simulink model "open_loop_model_compare"  (R2022b)
settings: Solver=ode45  StartTime=0.0  StopTime=5  FixedStep=0.01  RelTol=1e-3  EnableMultiTasking=on
settings Model: Creator=cpmcclel  LastModifiedBy=kaiwe
settings SolverCC: AlgebraicLoopSolver=TrustRegion
settings DataIOCC: LimitDataPoints=on  SaveFormat=Array  ReturnWorkspaceOutputs=off
settings OptimizationCC: LifeSpan=inf
settings DebuggingCC: SolverPrmCheckMsg=warning  UnconnectedInputMsg=warning  UnconnectedOutputMsg=warning  UnconnectedLineMsg=warning  SFUnexpectedBacktrackingDiag=warning  SFNoUnconditionalDefaultTransitionDiag=warning  SFExecutionAtInitializationDiag=none  SFMachineParentedDataDiag=warning  ArithmeticOperatorsInVariantConditions=warning
settings HardwareCC: ProdBitPerPointer=32  ProdBitPerSizeT=32  ProdBitPerPtrDiffT=32  ProdLargestAtomicFloat=None  ProdIntDivRoundTo=Undefined  ProdEndianess=Unspecified  ProdWordSize=32  ProdHWDeviceType=32-bit Generic
settings ModelReferenceCC: EnableRefExpFcnMdlSchedulingChecks=on  PropagateSignalLabelsOutOfModel=off
settings SFSimCC: SimUseLocalCustomCode=off  CustomCodeUndefinedFunction=UseInterfaceOnly
settings RTWCC: RTWUseLocalCustomCode=off
settings CodeAppCC: StateflowObjectComments=on
settings GRTTargetCC: TargetLangStandard=C89/C90 (ANSI)
settings ConfigComp: CovMetricSettings=dw  CovSaveCumulativeToWorkspaceVar=on  CovSaveSingleToWorkspaceVar=on  CovExternalEMLEnable=off  CovSFcnEnable=off

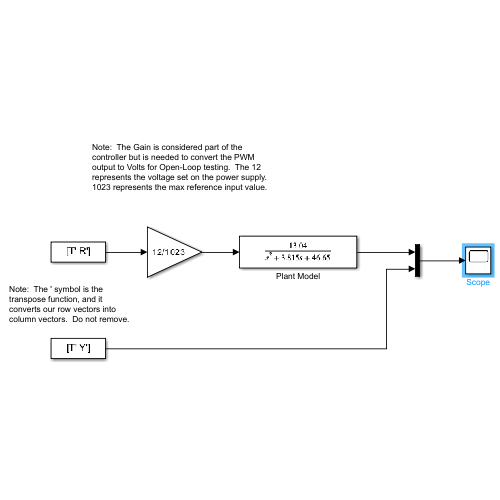
[thumbnail: Simulink's stored preview of the top-level diagram]
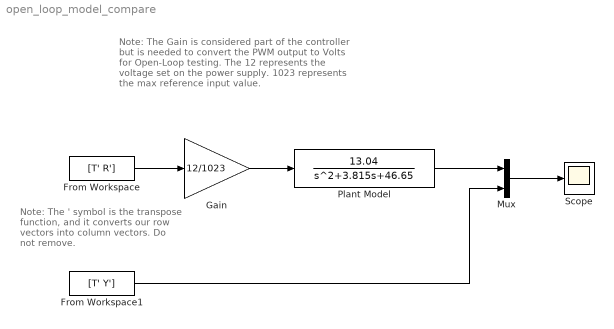
== system open_loop_model_compare ==
  note: Note: The Gain is considered part of the controller but is needed to convert the PWM output to Volts for Open-Loop testing. The 12 represents the voltage set on the power supply. 1023 represents the max reference input value.
  note: Note: The ' symbol is the transpose function, and it converts our row vectors into column vectors. Do not remove.
  From Workspace : FromWorkspace  VariableName=[T' R']  SampleTime=.01
  From Workspace1 : FromWorkspace  VariableName=[T' Y']  SampleTime=-1
  Gain : Gain  Gain=12/1023
  Mux : Mux  Inputs=2
  Plant Model : TransferFcn  Numerator=[13.04]  Denominator=[1 3.815 46.65]
  Scope : Scope
  wires:
  From Workspace/1 -> Gain/1
  Mux/1 -> Scope/1
  From Workspace1/1 -> Mux/2
  Plant Model/1 -> Mux/1
  Gain/1 -> Plant Model/1
